simulink model "xhand_sphere_tube_r50_v3"  (R2022b)
settings: Solver=VariableStepAuto  StartTime=0.0  StopTime=5  RelTol=1e-3
InitFcn:
  | clc;
  | clear;
  | addpath('H:\研究生\新建文件夹\xhand\meshes');
  | radium=0.055
  | global flag_gravity;
  | flag_gravity=0;
undefined symbols (not defined in the file): X, Y, Z
libraries: sm_lib x125, nesl_utility x27, Contact_Forces_Lib x26
(part 4 of 5)

== system xhand_sphere_tube_r50_v3/Subsystem/t5 ==
  Inertia : sm_lib/Body Elements/Inertia  InertiaType=Custom  Mass=0.00236998990932685  MassUnits=kg  CenterOfMass=[0, 0, 0]  CenterOfMassUnits=m  MomentsOfInertia=[1.05976671520843e-07, 4.46871056730638e-08, 1.03242419674807e-07]  MomentsOfInertiaUnits=kg*m^2  ProductsOfInertia=[1.03418479605301e-08, -7.1242901669066e-14, 2.53163731637035e-13]  ProductsOfInertiaUnits=kg*m^2  GraphicType=None  MarkerShape=Inertia  MarkerSize=20  GraphicVisPropType=SimpleVisualProperties  GraphicDiffuseColor=[0.5 0.5 0.5]  GraphicSpecularColor=[0.5 0.5 0.5 1.0]  GraphicAmbientColor=[0.15 0.15 0.15 1.0]  GraphicEmissiveColor=[0.0 0.0 0.0 1.0]  GraphicShininess=75  GraphicOpacity=1.0
  InertiaOriginTransform : sm_lib/Frames and Transforms/Rigid Transform  TranslationMethod=Cartesian  TranslationStandardOffset=0  TranslationLengthUnit=m  TranslationStandardAxis=+Z  TranslationCartesianOffset=[-0.00194844009875494, 0.015770875203899, -0.00157561387804256]  TranslationROffset=0  TranslationROffsetUnits=m  TranslationZOffset=0  TranslationZOffsetUnits=m  TranslationThetaOffset=0  TranslationThetaOffsetUnits=deg  RotationMethod=RotationSequence  RotationAngleUnits=deg  RotationStandardAxis=+Z  RotationAngle=0.0  RotationArbitraryAxis=[0 0 1]  FollAlignAxisA=+X  BaseAlignAxisA=+Y  FollAlignAxisB=+Y  BaseAlignAxisB=+Z  RotationSequenceAxes=BaseAxes  RotationSequence=XYZ  RotationSequenceAngles=[0, 0, 0]  RotationSequenceAnglesUnits=rad  RotationMatrix=[1 0 0; 0 1 0; 0 0 1]  Quaternion=[1 0 0 0]
  ReferenceFrame : sm_lib/Frames and Transforms/Reference Frame
  Visual : sm_lib/Body Elements/File Solid  ExtGeomFileName=xhand/meshes/t2.STL  UnitType=Custom  ExtGeomFileUnits=m  StepReaderType=HEX  ExportConvexHullGeometry=off  InertiaType=Custom  Mass=0  MassUnits=kg  CenterOfMass=[0, 0, 0]  CenterOfMassUnits=m  MomentsOfInertia=[0, 0, 0]  MomentsOfInertiaUnits=kg*m^2  ProductsOfInertia=[0, 0, 0]  ProductsOfInertiaUnits=kg*m^2  BasedOnType=DensityFromFile  Density=1000  DensityUnits=kg/m^3  DoExposeReferenceFrame=on  SerializedFrames=<Frames/>  GraphicType=FromGeometry  MarkerShape=Sphere  MarkerSize=10  GraphicVisPropType=SimpleVisualProperties  GraphicDiffuseColor=[1, 1, 1]  GraphicSpecularColor=[0.5 0.5 0.5 1.0]  GraphicAmbientColor=[0.15 0.15 0.15 1.0]  GraphicEmissiveColor=[0.0 0.0 0.0 1.0]  GraphicShininess=75  GraphicOpacity=1
  VisualOriginTransform : sm_lib/Frames and Transforms/Rigid Transform  TranslationMethod=Cartesian  TranslationStandardOffset=0  TranslationLengthUnit=m  TranslationStandardAxis=+Z  TranslationCartesianOffset=[0, 0, 0]  TranslationROffset=0  TranslationROffsetUnits=m  TranslationZOffset=0  TranslationZOffsetUnits=m  TranslationThetaOffset=0  TranslationThetaOffsetUnits=deg  RotationMethod=RotationSequence  RotationAngleUnits=deg  RotationStandardAxis=+Z  RotationAngle=0.0  RotationArbitraryAxis=[0 0 1]  FollAlignAxisA=+X  BaseAlignAxisA=+Y  FollAlignAxisB=+Y  BaseAlignAxisB=+Z  RotationSequenceAxes=BaseAxes  RotationSequence=XYZ  RotationSequenceAngles=[0, 0, 0]  RotationSequenceAnglesUnits=rad  RotationMatrix=[1 0 0; 0 1 0; 0 0 1]  Quaternion=[1 0 0 0]
  t2_AxisInvTransform : sm_lib/Frames and Transforms/Rigid Transform  TranslationMethod=Cartesian  TranslationStandardOffset=0  TranslationLengthUnit=m  TranslationStandardAxis=+Z  TranslationCartesianOffset=[0, 0, 0]  TranslationROffset=0  TranslationROffsetUnits=m  TranslationZOffset=0  TranslationZOffsetUnits=m  TranslationThetaOffset=0  TranslationThetaOffsetUnits=deg  RotationMethod=ArbitraryAxis  RotationAngleUnits=rad  RotationStandardAxis=+Z  RotationAngle=1.570796326794897  RotationArbitraryAxis=[-0, -1, 0]  FollAlignAxisA=+X  BaseAlignAxisA=+Y  FollAlignAxisB=+Y  BaseAlignAxisB=+Z  RotationSequenceAxes=FollowerAxes  RotationSequence=XYX  RotationSequenceAngles=[0 0 0]  RotationSequenceAnglesUnits=deg  RotationMatrix=[1 0 0; 0 1 0; 0 0 1]  Quaternion=[1 0 0 0]
  F : PMIOPort  Side=Left
  t2 : PMIOPort  Port=2  Side=Left
  connections:
  Inertia/RConn1 -- InertiaOriginTransform/RConn1
  ReferenceFrame/RConn1 -- InertiaOriginTransform/LConn1 -- VisualOriginTransform/LConn1 -- t2_AxisInvTransform/LConn1
  Visual/RConn1 -- t2/RConn1 -- VisualOriginTransform/RConn1
  t2_AxisInvTransform/RConn1 -- F/RConn1

== system xhand_sphere_tube_r50_v3/Subsystem14/Subsystem10 ==
  Bus Selector10 : BusSelector  OutputSignals=Normal Force
  Bus Selector26 : BusSelector  OutputSignals=Frame Sep.x,Frame Sep.y,Frame Sep.z
  Rigid Transform10 : sm_lib/Frames and Transforms/Rigid Transform  TranslationMethod=Cartesian  TranslationStandardOffset=0  TranslationLengthUnit=m  TranslationStandardAxis=+Z  TranslationCartesianOffset=[0.0020 0.044/2 -0.000]  TranslationROffset=0  TranslationROffsetUnits=m  TranslationZOffset=0  TranslationZOffsetUnits=m  TranslationThetaOffset=0  TranslationThetaOffsetUnits=deg  RotationMethod=StandardAxis  RotationAngleUnits=deg  RotationStandardAxis=+X  RotationAngle=90.0  RotationArbitraryAxis=[0 0 1]  FollAlignAxisA=+X  BaseAlignAxisA=+Y  FollAlignAxisB=+Y  BaseAlignAxisB=+Z  RotationSequenceAxes=FollowerAxes  RotationSequence=XYX  RotationSequenceAngles=[0 0 0]  RotationSequenceAnglesUnits=deg  RotationMatrix=[1 0 0; 0 1 0; 0 0 1]  Quaternion=[1 0 0 0]
  Sphere to Plane Force7 : Contact_Forces_Lib/3D/Sphere to Plane Force  sphere_rad=0.00000000001  plane_lenx=0.00000000001  plane_leny=0.00000000001  plane_depth=0.00000000001  force_law=Nonlinear  k_contact=10e1  b_contact=10^0.5  pen_full_damp_F=1e-4  pen_exponent=1  custom_param_1=1  custom_param_2=1  friction_law=Stick-Slip Continuous  mu_kinetic=0.3  mu_static=0.5  v_thr=0.02  vis_on=on  vis_opc_en=0  vis_len_plaBz=0.0001  vis_clr=[0.9 0.2 0.2]  vis_opc=0.7
  Sphere to Tube Force8 : Contact_Forces_Lib/3D/Sphere to Tube Force  radius_sphere=radium  radius_tube=0.013/4  d_tube=0.0135/2  l_tube=0.042  active_angle=[-180 180]  force_law=Nonlinear  k_contact=1e3  b_contact=1e1  pen_full_damp_F=1e-4  pen_exponent=1  custom_param_1=1  custom_param_2=1  friction_law=Stick-Slip Continuous  mu_kinetic=0.5  mu_static=0.7  v_thr=0.001  vis_on=off  vis_opc_en=0  vis_len_tubBx=0.225*0.02  vis_clr=[0.9 0.2 0.2]  vis_opc=0.7
      settings: SourceProductName=Simscape Multibody Contact Forces Library
  mmcp : PMIOPort  Side=Right
  SphF : PMIOPort  Port=2  Side=Left
  <Normal Force> : Outport
  <x> : Outport  Port=2
  <y> : Outport  Port=3
  <z> : Outport  Port=4
  wires:
  Bus Selector26/1 -> <x>/1  "<x>"
  Bus Selector10/1 -> <Normal Force>/1  "<Normal Force>"
  Sphere to Tube Force8/1 -> Bus Selector10/1
  Sphere to Plane Force7/1 -> Bus Selector26/1
  Bus Selector26/2 -> <y>/1  "<y>"
  Bus Selector26/3 -> <z>/1  "<z>"
  connections:
  Rigid Transform10/LConn1 -- mmcp/RConn1 -- Sphere to Plane Force7/RConn1
  Sphere to Tube Force8/RConn1 -- Rigid Transform10/RConn1
  Sphere to Tube Force8/LConn1 -- Sphere to Plane Force7/LConn1 -- SphF/RConn1

== system xhand_sphere_tube_r50_v3/Subsystem14/Subsystem11 ==
  Bus Selector11 : BusSelector  OutputSignals=Normal Force
  Bus Selector39 : BusSelector  OutputSignals=Frame Sep.x,Frame Sep.y,Frame Sep.z
  Rigid Transform11 : sm_lib/Frames and Transforms/Rigid Transform  TranslationMethod=Cartesian  TranslationStandardOffset=0  TranslationLengthUnit=m  TranslationStandardAxis=+Z  TranslationCartesianOffset=[0.002 0.038/2 -0.000]  TranslationROffset=0  TranslationROffsetUnits=m  TranslationZOffset=0  TranslationZOffsetUnits=m  TranslationThetaOffset=0  TranslationThetaOffsetUnits=deg  RotationMethod=StandardAxis  RotationAngleUnits=deg  RotationStandardAxis=+X  RotationAngle=90.0  RotationArbitraryAxis=[0 0 1]  FollAlignAxisA=+X  BaseAlignAxisA=+Y  FollAlignAxisB=+Y  BaseAlignAxisB=+Z  RotationSequenceAxes=FollowerAxes  RotationSequence=XYX  RotationSequenceAngles=[0 0 0]  RotationSequenceAnglesUnits=deg  RotationMatrix=[1 0 0; 0 1 0; 0 0 1]  Quaternion=[1 0 0 0]
  Sphere to Plane Force6 : Contact_Forces_Lib/3D/Sphere to Plane Force  sphere_rad=radium+0.001  plane_lenx=0.006*2  plane_leny=0.031*2  plane_depth=0.0124/2*0.4  force_law=Nonlinear  k_contact=10e1  b_contact=10^0.5  pen_full_damp_F=1e-4  pen_exponent=1  custom_param_1=1  custom_param_2=1  friction_law=Stick-Slip Continuous  mu_kinetic=0.5  mu_static=0.7  v_thr=0.05  vis_on=off  vis_opc_en=0  vis_len_plaBz=0.0001  vis_clr=[0.9 0.2 0.2]  vis_opc=0.7
  Sphere to Tube Force9 : Contact_Forces_Lib/3D/Sphere to Tube Force  radius_sphere=radium  radius_tube=0.0135/4  d_tube=0.0135/2  l_tube=0.038  active_angle=[-180 180]  force_law=Nonlinear  k_contact=1e3  b_contact=1e1  pen_full_damp_F=1e-4  pen_exponent=1  custom_param_1=1  custom_param_2=1  friction_law=Stick-Slip Continuous  mu_kinetic=0.5  mu_static=0.7  v_thr=0.001  vis_on=off  vis_opc_en=0  vis_len_tubBx=0.225*0.02  vis_clr=[0.9 0.2 0.2]  vis_opc=0.7
      settings: SourceProductName=Simscape Multibody Contact Forces Library
  imcp : PMIOPort  Side=Right
  SphF : PMIOPort  Port=2  Side=Left
  <Normal Force> : Outport
  <x> : Outport  Port=2
  <y> : Outport  Port=3
  <z> : Outport  Port=4
  wires:
  Sphere to Tube Force9/1 -> Bus Selector11/1
  Bus Selector39/1 -> <x>/1  "<x>"
  Sphere to Plane Force6/1 -> Bus Selector39/1
  Bus Selector11/1 -> <Normal Force>/1  "<Normal Force>"
  Bus Selector39/2 -> <y>/1  "<y>"
  Bus Selector39/3 -> <z>/1  "<z>"
  connections:
  Sphere to Tube Force9/LConn1 -- Sphere to Plane Force6/LConn1 -- SphF/RConn1
  Sphere to Tube Force9/RConn1 -- Rigid Transform11/RConn1
  Rigid Transform11/LConn1 -- imcp/RConn1 -- Sphere to Plane Force6/RConn1

== system xhand_sphere_tube_r50_v3/Subsystem14/Subsystem12 ==
  Bus Selector18 : BusSelector  OutputSignals=Normal Force
  Bus Selector38 : BusSelector  OutputSignals=Frame Sep.x,Frame Sep.y,Frame Sep.z
  Rigid Transform3 : sm_lib/Frames and Transforms/Rigid Transform  TranslationMethod=Cartesian  TranslationStandardOffset=0  TranslationLengthUnit=m  TranslationStandardAxis=+Z  TranslationCartesianOffset=[0.002 0.04/2 0.0005]  TranslationROffset=0  TranslationROffsetUnits=m  TranslationZOffset=0  TranslationZOffsetUnits=m  TranslationThetaOffset=0  TranslationThetaOffsetUnits=deg  RotationMethod=StandardAxis  RotationAngleUnits=deg  RotationStandardAxis=+X  RotationAngle=90.0  RotationArbitraryAxis=[0 0 1]  FollAlignAxisA=+X  BaseAlignAxisA=+Y  FollAlignAxisB=+Y  BaseAlignAxisB=+Z  RotationSequenceAxes=FollowerAxes  RotationSequence=XYX  RotationSequenceAngles=[0 0 0]  RotationSequenceAnglesUnits=deg  RotationMatrix=[1 0 0; 0 1 0; 0 0 1]  Quaternion=[1 0 0 0]
  Sphere to Plane Force10 : Contact_Forces_Lib/3D/Sphere to Plane Force  sphere_rad=0.0000000000001  plane_lenx=0.0000000000001  plane_leny=0.0000000000001  plane_depth=0.0000000000001  force_law=Nonlinear  k_contact=10^3  b_contact=10^1  pen_full_damp_F=1e-4  pen_exponent=1  custom_param_1=1  custom_param_2=1  friction_law=Stick-Slip Continuous  mu_kinetic=0.5  mu_static=0.7  v_thr=0.05  vis_on=on  vis_opc_en=0  vis_len_plaBz=0.0001  vis_clr=[0.9 0.2 0.2]  vis_opc=0.7
  Sphere to Tube Force : Contact_Forces_Lib/3D/Sphere to Tube Force  radius_sphere=radium+0.001  radius_tube=0.0126/4  d_tube=0.0126/2  l_tube=0.033  active_angle=[-180 180]  force_law=Nonlinear  k_contact=1e3  b_contact=1e1  pen_full_damp_F=1e-4  pen_exponent=1  custom_param_1=1  custom_param_2=1  friction_law=Stick-Slip Continuous  mu_kinetic=0.5  mu_static=0.7  v_thr=0.001  vis_on=off  vis_opc_en=0  vis_len_tubBx=0.225*0.02  vis_clr=[0.9 0.2 0.2]  vis_opc=0.7
      settings: SourceProductName=Simscape Multibody Contact Forces Library
  tmcp : PMIOPort  Side=Right
  SphF : PMIOPort  Port=2  Side=Left
  <Normal Force> : Outport
  <x> : Outport  Port=2
  <y> : Outport  Port=3
  <z> : Outport  Port=4
  wires:
  Sphere to Plane Force10/1 -> Bus Selector38/1
  Sphere to Tube Force/1 -> Bus Selector18/1
  Bus Selector18/1 -> <Normal Force>/1  "<Normal Force>"
  Bus Selector38/3 -> <z>/1  "<z>"
  Bus Selector38/2 -> <y>/1  "<y>"
  Bus Selector38/1 -> <x>/1  "<x>"
  connections:
  Sphere to Tube Force/RConn1 -- Rigid Transform3/RConn1
  Rigid Transform3/LConn1 -- tmcp/RConn1 -- Sphere to Plane Force10/RConn1
  Sphere to Tube Force/LConn1 -- Sphere to Plane Force10/LConn1 -- SphF/RConn1

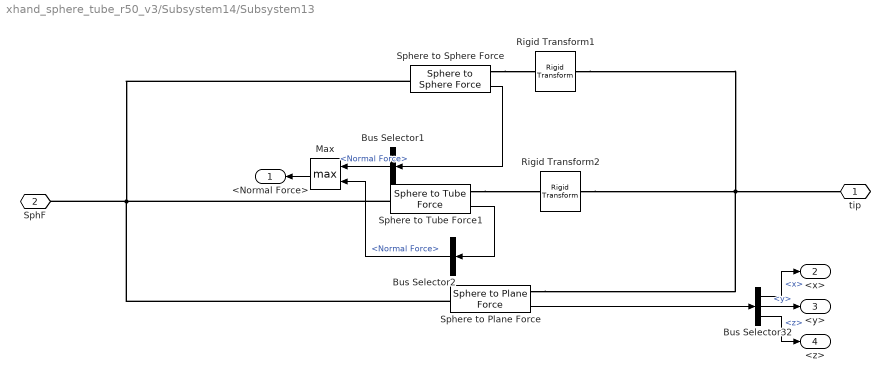
== system xhand_sphere_tube_r50_v3/Subsystem14/Subsystem13 ==
  Bus Selector1 : BusSelector  OutputSignals=Normal Force
  Bus Selector2 : BusSelector  OutputSignals=Normal Force
  Bus Selector32 : BusSelector  OutputSignals=Frame Sep.x,Frame Sep.y,Frame Sep.z
  Max : MinMax  Function=max  Inputs=2
  Rigid Transform1 : sm_lib/Frames and Transforms/Rigid Transform  TranslationMethod=Cartesian  TranslationStandardOffset=0  TranslationLengthUnit=m  TranslationStandardAxis=+Z  TranslationCartesianOffset=[-0.0019 0.053/2 -0.0022]  TranslationROffset=0  TranslationROffsetUnits=m  TranslationZOffset=0  TranslationZOffsetUnits=m  TranslationThetaOffset=0  TranslationThetaOffsetUnits=deg  RotationMethod=StandardAxis  RotationAngleUnits=deg  RotationStandardAxis=+X  RotationAngle=90.0  RotationArbitraryAxis=[0 0 1]  FollAlignAxisA=+X  BaseAlignAxisA=+Y  FollAlignAxisB=+Y  BaseAlignAxisB=+Z  RotationSequenceAxes=FollowerAxes  RotationSequence=XYX  RotationSequenceAngles=[0 0 0]  RotationSequenceAnglesUnits=deg  RotationMatrix=[1 0 0; 0 1 0; 0 0 1]  Quaternion=[1 0 0 0]
  Rigid Transform2 : sm_lib/Frames and Transforms/Rigid Transform  TranslationMethod=Cartesian  TranslationStandardOffset=0  TranslationLengthUnit=m  TranslationStandardAxis=+Z  TranslationCartesianOffset=[-0.0019 0.03/2 -0.003]  TranslationROffset=0  TranslationROffsetUnits=m  TranslationZOffset=0  TranslationZOffsetUnits=m  TranslationThetaOffset=0  TranslationThetaOffsetUnits=deg  RotationMethod=StandardAxis  RotationAngleUnits=deg  RotationStandardAxis=+X  RotationAngle=90.0  RotationArbitraryAxis=[0 0 1]  FollAlignAxisA=+X  BaseAlignAxisA=+Y  FollAlignAxisB=+Y  BaseAlignAxisB=+Z  RotationSequenceAxes=FollowerAxes  RotationSequence=XYX  RotationSequenceAngles=[0 0 0]  RotationSequenceAnglesUnits=deg  RotationMatrix=[1 0 0; 0 1 0; 0 0 1]  Quaternion=[1 0 0 0]
  Sphere to Plane Force : Contact_Forces_Lib/3D/Sphere to Plane Force  sphere_rad=0.0000000000001  plane_lenx=0.0000000000001  plane_leny=0.0000000000001  plane_depth=0.0000000000001  force_law=Nonlinear  k_contact=10^3  b_contact=10^1  pen_full_damp_F=1e-4  pen_exponent=1  custom_param_1=1  custom_param_2=1  friction_law=Stick-Slip Continuous  mu_kinetic=0.5  mu_static=0.7  v_thr=0.05  vis_on=off  vis_opc_en=0  vis_len_plaBz=0.0001  vis_clr=[0.9 0.2 0.2]  vis_opc=0.7
  Sphere to Sphere Force : Contact_Forces_Lib/3D/Sphere to Sphere Force  sphB_rad=0.0058  sphF_rad=radium  force_law=Nonlinear  k_contact=1e4  b_contact=1e2  pen_full_damp_F=1e-4  pen_exponent=1  custom_param_1=1  custom_param_2=1  friction_law=Stick-Slip Continuous  mu_kinetic=0.6  mu_static=0.7  v_thr=0.001  vis_on=off  vis_opc_en=0  vis_clr=[0.9 0.2 0.2]  vis_opc=0.7
      settings: SourceProductName=Simscape Multibody Contact Forces Library
  Sphere to Tube Force1 : Contact_Forces_Lib/3D/Sphere to Tube Force  radius_sphere=radium+0.00  radius_tube=0.012/4  d_tube=0.012/2  l_tube=0.03  active_angle=[-180 180]  force_law=Nonlinear  k_contact=1e4  b_contact=1e2  pen_full_damp_F=1e-4  pen_exponent=1  custom_param_1=1  custom_param_2=1  friction_law=Stick-Slip Continuous  mu_kinetic=0.6  mu_static=0.7  v_thr=0.001  vis_on=off  vis_opc_en=0  vis_len_tubBx=0.225*0.02  vis_clr=[0.9 0.2 0.2]  vis_opc=0.7
      settings: SourceProductName=Simscape Multibody Contact Forces Library
  tip : PMIOPort  Side=Right
  SphF : PMIOPort  Port=2  Side=Left
  <Normal Force> : Outport
  <x> : Outport  Port=2
  <y> : Outport  Port=3
  <z> : Outport  Port=4
  wires:
  Bus Selector32/1 -> <x>/1  "<x>"
  Bus Selector32/2 -> <y>/1  "<y>"
  Sphere to Plane Force/1 -> Bus Selector32/1
  Sphere to Tube Force1/1 -> Bus Selector2/1
  Bus Selector32/3 -> <z>/1  "<z>"
  Bus Selector1/1 -> Max/1  "<Normal Force>"
  Max/1 -> <Normal Force>/1
  Bus Selector2/1 -> Max/2  "<Normal Force>"
  Sphere to Sphere Force/1 -> Bus Selector1/1
  connections:
  Sphere to Tube Force1/RConn1 -- Rigid Transform2/RConn1
  Rigid Transform2/LConn1 -- Rigid Transform1/LConn1 -- tip/RConn1 -- Sphere to Plane Force/RConn1
  Sphere to Tube Force1/LConn1 -- Sphere to Sphere Force/LConn1 -- Sphere to Plane Force/LConn1 -- SphF/RConn1
  Sphere to Sphere Force/RConn1 -- Rigid Transform1/RConn1

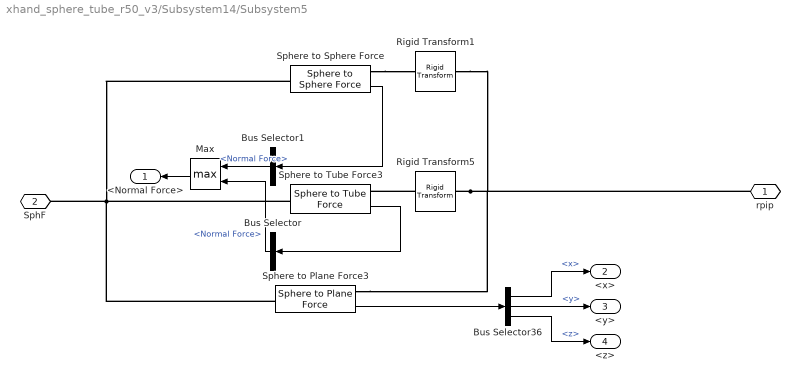
== system xhand_sphere_tube_r50_v3/Subsystem14/Subsystem5 ==
  Bus Selector : BusSelector  OutputSignals=Normal Force
  Bus Selector1 : BusSelector  OutputSignals=Normal Force
  Bus Selector36 : BusSelector  OutputSignals=Frame Sep.x,Frame Sep.y,Frame Sep.z
  Max : MinMax  Function=max  Inputs=2
  Rigid Transform1 : sm_lib/Frames and Transforms/Rigid Transform  TranslationMethod=Cartesian  TranslationStandardOffset=0  TranslationLengthUnit=m  TranslationStandardAxis=+Z  TranslationCartesianOffset=[-0.002 0.0525/2 -0.0018]  TranslationROffset=0  TranslationROffsetUnits=m  TranslationZOffset=0  TranslationZOffsetUnits=m  TranslationThetaOffset=0  TranslationThetaOffsetUnits=deg  RotationMethod=StandardAxis  RotationAngleUnits=deg  RotationStandardAxis=+X  RotationAngle=90.0  RotationArbitraryAxis=[0 0 1]  FollAlignAxisA=+X  BaseAlignAxisA=+Y  FollAlignAxisB=+Y  BaseAlignAxisB=+Z  RotationSequenceAxes=FollowerAxes  RotationSequence=XYX  RotationSequenceAngles=[0 0 0]  RotationSequenceAnglesUnits=deg  RotationMatrix=[1 0 0; 0 1 0; 0 0 1]  Quaternion=[1 0 0 0]
  Rigid Transform5 : sm_lib/Frames and Transforms/Rigid Transform  TranslationMethod=Cartesian  TranslationStandardOffset=0  TranslationLengthUnit=m  TranslationStandardAxis=+Z  TranslationCartesianOffset=[-0.0019 0.032/2 -0.0018]  TranslationROffset=0  TranslationROffsetUnits=m  TranslationZOffset=0  TranslationZOffsetUnits=m  TranslationThetaOffset=0  TranslationThetaOffsetUnits=deg  RotationMethod=StandardAxis  RotationAngleUnits=deg  RotationStandardAxis=+X  RotationAngle=90.0  RotationArbitraryAxis=[0 0 1]  FollAlignAxisA=+X  BaseAlignAxisA=+Y  FollAlignAxisB=+Y  BaseAlignAxisB=+Z  RotationSequenceAxes=FollowerAxes  RotationSequence=XYX  RotationSequenceAngles=[0 0 0]  RotationSequenceAnglesUnits=deg  RotationMatrix=[1 0 0; 0 1 0; 0 0 1]  Quaternion=[1 0 0 0]
  Sphere to Plane Force3 : Contact_Forces_Lib/3D/Sphere to Plane Force  sphere_rad=0.00000000001  plane_lenx=0.00000000001  plane_leny=0.00000000001  plane_depth=0.00000000001  force_law=Nonlinear  k_contact=10e1  b_contact=10^0.5  pen_full_damp_F=1e-4  pen_exponent=1  custom_param_1=1  custom_param_2=1  friction_law=Stick-Slip Continuous  mu_kinetic=0.5  mu_static=0.7  v_thr=0.05  vis_on=off  vis_opc_en=0  vis_len_plaBz=0.0001  vis_clr=[0.9 0.2 0.2]  vis_opc=0.7
  Sphere to Sphere Force : Contact_Forces_Lib/3D/Sphere to Sphere Force  sphB_rad=0.006  sphF_rad=radium  force_law=Nonlinear  k_contact=1e4  b_contact=1e2  pen_full_damp_F=1e-4  pen_exponent=1  custom_param_1=1  custom_param_2=1  friction_law=Stick-Slip Continuous  mu_kinetic=0.6  mu_static=0.7  v_thr=0.001  vis_on=off  vis_opc_en=0  vis_clr=[0.9 0.2 0.2]  vis_opc=0.7
      settings: SourceProductName=Simscape Multibody Contact Forces Library
  Sphere to Tube Force3 : Contact_Forces_Lib/3D/Sphere to Tube Force  radius_sphere=radium  radius_tube=0.011/4  d_tube=0.012/2  l_tube=0.032  active_angle=[-180 180]  force_law=Nonlinear  k_contact=1e4  b_contact=1e2  pen_full_damp_F=1e-4  pen_exponent=1  custom_param_1=1  custom_param_2=1  friction_law=Stick-Slip Continuous  mu_kinetic=0.6  mu_static=0.7  v_thr=0.001  vis_on=off  vis_opc_en=0  vis_len_tubBx=0.225*0.02  vis_clr=[0.9 0.2 0.2]  vis_opc=0.7
      settings: SourceProductName=Simscape Multibody Contact Forces Library
  rpip : PMIOPort  Side=Right
  SphF : PMIOPort  Port=2  Side=Left
  <Normal Force> : Outport
  <x> : Outport  Port=2
  <y> : Outport  Port=3
  <z> : Outport  Port=4
  wires:
  Sphere to Tube Force3/1 -> Bus Selector/1
  Sphere to Plane Force3/1 -> Bus Selector36/1
  Bus Selector36/2 -> <y>/1  "<y>"
  Bus Selector36/3 -> <z>/1  "<z>"
  Bus Selector36/1 -> <x>/1  "<x>"
  Sphere to Sphere Force/1 -> Bus Selector1/1
  Max/1 -> <Normal Force>/1
  Bus Selector/1 -> Max/2  "<Normal Force>"
  Bus Selector1/1 -> Max/1  "<Normal Force>"
  connections:
  Rigid Transform5/LConn1 -- Rigid Transform1/LConn1 -- rpip/RConn1 -- Sphere to Plane Force3/RConn1
  Rigid Transform5/RConn1 -- Sphere to Tube Force3/RConn1
  Sphere to Tube Force3/LConn1 -- Sphere to Sphere Force/LConn1 -- Sphere to Plane Force3/LConn1 -- SphF/RConn1
  Sphere to Sphere Force/RConn1 -- Rigid Transform1/RConn1

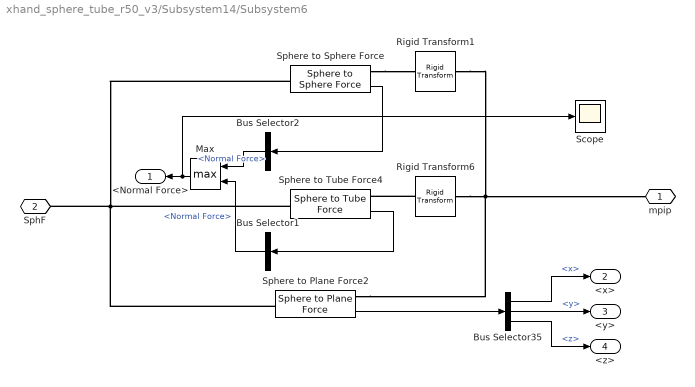
== system xhand_sphere_tube_r50_v3/Subsystem14/Subsystem6 ==
  Bus Selector1 : BusSelector  OutputSignals=Normal Force
  Bus Selector2 : BusSelector  OutputSignals=Normal Force
  Bus Selector35 : BusSelector  OutputSignals=Frame Sep.x,Frame Sep.y,Frame Sep.z
  Max : MinMax  Function=max  Inputs=2
  Rigid Transform1 : sm_lib/Frames and Transforms/Rigid Transform  TranslationMethod=Cartesian  TranslationStandardOffset=0  TranslationLengthUnit=m  TranslationStandardAxis=+Z  TranslationCartesianOffset=[-0.0019 0.0705/2 -0.0019]  TranslationROffset=0  TranslationROffsetUnits=m  TranslationZOffset=0  TranslationZOffsetUnits=m  TranslationThetaOffset=0  TranslationThetaOffsetUnits=deg  RotationMethod=StandardAxis  RotationAngleUnits=deg  RotationStandardAxis=+X  RotationAngle=90.0  RotationArbitraryAxis=[0 0 1]  FollAlignAxisA=+X  BaseAlignAxisA=+Y  FollAlignAxisB=+Y  BaseAlignAxisB=+Z  RotationSequenceAxes=FollowerAxes  RotationSequence=XYX  RotationSequenceAngles=[0 0 0]  RotationSequenceAnglesUnits=deg  RotationMatrix=[1 0 0; 0 1 0; 0 0 1]  Quaternion=[1 0 0 0]
  Rigid Transform6 : sm_lib/Frames and Transforms/Rigid Transform  TranslationMethod=Cartesian  TranslationStandardOffset=0  TranslationLengthUnit=m  TranslationStandardAxis=+Z  TranslationCartesianOffset=[-0.0019 0.038/2 -0.0018]  TranslationROffset=0  TranslationROffsetUnits=m  TranslationZOffset=0  TranslationZOffsetUnits=m  TranslationThetaOffset=0  TranslationThetaOffsetUnits=deg  RotationMethod=StandardAxis  RotationAngleUnits=deg  RotationStandardAxis=+X  RotationAngle=90.0  RotationArbitraryAxis=[0 0 1]  FollAlignAxisA=+X  BaseAlignAxisA=+Y  FollAlignAxisB=+Y  BaseAlignAxisB=+Z  RotationSequenceAxes=FollowerAxes  RotationSequence=XYX  RotationSequenceAngles=[0 0 0]  RotationSequenceAnglesUnits=deg  RotationMatrix=[1 0 0; 0 1 0; 0 0 1]  Quaternion=[1 0 0 0]
  Scope : Scope
  Sphere to Plane Force2 : Contact_Forces_Lib/3D/Sphere to Plane Force  sphere_rad=0.00000000001  plane_lenx=0.00000000001  plane_leny=0.00000000001  plane_depth=0.00000000001  force_law=Nonlinear  k_contact=10e3  b_contact=10^1  pen_full_damp_F=1e-4  pen_exponent=1  custom_param_1=1  custom_param_2=1  friction_law=Stick-Slip Continuous  mu_kinetic=0.3  mu_static=0.5  v_thr=0.02  vis_on=off  vis_opc_en=0  vis_len_plaBz=0.0001  vis_clr=[0.9 0.2 0.2]  vis_opc=0.7
  Sphere to Sphere Force : Contact_Forces_Lib/3D/Sphere to Sphere Force  sphB_rad=0.0053  sphF_rad=radium  force_law=Nonlinear  k_contact=1e4  b_contact=1e2  pen_full_damp_F=1e-4  pen_exponent=1  custom_param_1=1  custom_param_2=1  friction_law=Stick-Slip Continuous  mu_kinetic=0.6  mu_static=0.7  v_thr=0.001  vis_on=off  vis_opc_en=0  vis_clr=[0.9 0.2 0.2]  vis_opc=0.7
      settings: SourceProductName=Simscape Multibody Contact Forces Library
  Sphere to Tube Force4 : Contact_Forces_Lib/3D/Sphere to Tube Force  radius_sphere=radium+0.00  radius_tube=0.0118/4  d_tube=0.01/2  l_tube=0.04  active_angle=[-180 180]  force_law=Nonlinear  k_contact=1e4  b_contact=1e2  pen_full_damp_F=1e-4  pen_exponent=1  custom_param_1=1  custom_param_2=1  friction_law=Stick-Slip Continuous  mu_kinetic=0.6  mu_static=0.7  v_thr=0.001  vis_on=off  vis_opc_en=0  vis_len_tubBx=0.225*0.02  vis_clr=[0.9 0.2 0.2]  vis_opc=0.7
      settings: SourceProductName=Simscape Multibody Contact Forces Library
  mpip : PMIOPort  Side=Right
  SphF : PMIOPort  Port=2  Side=Left
  <Normal Force> : Outport
  <x> : Outport  Port=2
  <y> : Outport  Port=3
  <z> : Outport  Port=4
  wires:
  Sphere to Plane Force2/1 -> Bus Selector35/1
  Sphere to Tube Force4/1 -> Bus Selector1/1
  Bus Selector35/2 -> <y>/1  "<y>"
  Bus Selector35/1 -> <x>/1  "<x>"
  Bus Selector35/3 -> <z>/1  "<z>"
  Sphere to Sphere Force/1 -> Bus Selector2/1
  Max/1 -> Scope/1, <Normal Force>/1
  Bus Selector1/1 -> Max/2  "<Normal Force>"
  Bus Selector2/1 -> Max/1  "<Normal Force>"
  connections:
  Sphere to Tube Force4/LConn1 -- Sphere to Plane Force2/LConn1 -- Sphere to Sphere Force/LConn1 -- SphF/RConn1
  Rigid Transform6/LConn1 -- Rigid Transform1/LConn1 -- mpip/RConn1 -- Sphere to Plane Force2/RConn1
  Rigid Transform6/RConn1 -- Sphere to Tube Force4/RConn1
  Sphere to Sphere Force/RConn1 -- Rigid Transform1/RConn1

== system xhand_sphere_tube_r50_v3/Subsystem14/Subsystem7 ==
  Bus Selector1 : BusSelector  OutputSignals=Normal Force
  Bus Selector29 : BusSelector  OutputSignals=Frame Sep.x,Frame Sep.y,Frame Sep.z
  Bus Selector3 : BusSelector  OutputSignals=Normal Force
  Max : MinMax  Function=max  Inputs=2
  Rigid Transform1 : sm_lib/Frames and Transforms/Rigid Transform  TranslationMethod=Cartesian  TranslationStandardOffset=0  TranslationLengthUnit=m  TranslationStandardAxis=+Z  TranslationCartesianOffset=[-0.0021 0.049/2 -0.0023]  TranslationROffset=0  TranslationROffsetUnits=m  TranslationZOffset=0  TranslationZOffsetUnits=m  TranslationThetaOffset=0  TranslationThetaOffsetUnits=deg  RotationMethod=StandardAxis  RotationAngleUnits=deg  RotationStandardAxis=+X  RotationAngle=90.0  RotationArbitraryAxis=[0 0 1]  FollAlignAxisA=+X  BaseAlignAxisA=+Y  FollAlignAxisB=+Y  BaseAlignAxisB=+Z  RotationSequenceAxes=FollowerAxes  RotationSequence=XYX  RotationSequenceAngles=[0 0 0]  RotationSequenceAnglesUnits=deg  RotationMatrix=[1 0 0; 0 1 0; 0 0 1]  Quaternion=[1 0 0 0]
  Rigid Transform7 : sm_lib/Frames and Transforms/Rigid Transform  TranslationMethod=Cartesian  TranslationStandardOffset=0  TranslationLengthUnit=m  TranslationStandardAxis=+Z  TranslationCartesianOffset=[-0.0021 0.030/2 -0.002]  TranslationROffset=0  TranslationROffsetUnits=m  TranslationZOffset=0  TranslationZOffsetUnits=m  TranslationThetaOffset=0  TranslationThetaOffsetUnits=deg  RotationMethod=StandardAxis  RotationAngleUnits=deg  RotationStandardAxis=+X  RotationAngle=90.0  RotationArbitraryAxis=[0 0 1]  FollAlignAxisA=+X  BaseAlignAxisA=+Y  FollAlignAxisB=+Y  BaseAlignAxisB=+Z  RotationSequenceAxes=FollowerAxes  RotationSequence=XYX  RotationSequenceAngles=[0 0 0]  RotationSequenceAnglesUnits=deg  RotationMatrix=[1 0 0; 0 1 0; 0 0 1]  Quaternion=[1 0 0 0]
  Sphere to Plane Force1 : Contact_Forces_Lib/3D/Sphere to Plane Force  sphere_rad=0.00000000001  plane_lenx=0.00000000001  plane_leny=0.00000000001  plane_depth=0.00000000001  force_law=Nonlinear  k_contact=10e1  b_contact=10^0.5  pen_full_damp_F=1e-4  pen_exponent=1  custom_param_1=1  custom_param_2=1  friction_law=Stick-Slip Continuous  mu_kinetic=0.5  mu_static=0.7  v_thr=0.05  vis_on=off  vis_opc_en=0  vis_len_plaBz=0.0001  vis_clr=[0.9 0.2 0.2]  vis_opc=0.7
  Sphere to Sphere Force : Contact_Forces_Lib/3D/Sphere to Sphere Force  sphB_rad=0.0058  sphF_rad=radium  force_law=Nonlinear  k_contact=1e4  b_contact=1e2  pen_full_damp_F=1e-4  pen_exponent=1  custom_param_1=1  custom_param_2=1  friction_law=Stick-Slip Continuous  mu_kinetic=0.6  mu_static=0.7  v_thr=0.001  vis_on=off  vis_opc_en=0  vis_clr=[0.9 0.2 0.2]  vis_opc=0.7
      settings: SourceProductName=Simscape Multibody Contact Forces Library
  Sphere to Tube Force5 : Contact_Forces_Lib/3D/Sphere to Tube Force  radius_sphere=radium  radius_tube=0.012/4  d_tube=0.012/2  l_tube=0.03  active_angle=[-180 180]  force_law=Nonlinear  k_contact=1e4  b_contact=1e2  pen_full_damp_F=1e-4  pen_exponent=1  custom_param_1=1  custom_param_2=1  friction_law=Stick-Slip Continuous  mu_kinetic=0.6  mu_static=0.7  v_thr=0.001  vis_on=off  vis_opc_en=0  vis_len_tubBx=0.225*0.02  vis_clr=[0.9 0.2 0.2]  vis_opc=0.7
      settings: SourceProductName=Simscape Multibody Contact Forces Library
  ipip : PMIOPort  Side=Right
  SphF : PMIOPort  Port=2  Side=Left
  <Normal Force> : Outport
  <x> : Outport  Port=2
  <y> : Outport  Port=3
  <z> : Outport  Port=4
  wires:
  Sphere to Tube Force5/1 -> Bus Selector3/1
  Sphere to Plane Force1/1 -> Bus Selector29/1
  Bus Selector3/1 -> Max/2  "<Normal Force>"
  Bus Selector29/3 -> <z>/1  "<z>"
  Bus Selector29/2 -> <y>/1  "<y>"
  Bus Selector29/1 -> <x>/1  "<x>"
  Sphere to Sphere Force/1 -> Bus Selector1/1
  Bus Selector1/1 -> Max/1  "<Normal Force>"
  Max/1 -> <Normal Force>/1
  connections:
  Sphere to Tube Force5/LConn1 -- Sphere to Plane Force1/LConn1 -- Sphere to Sphere Force/LConn1 -- SphF/RConn1
  Rigid Transform7/RConn1 -- Sphere to Tube Force5/RConn1
  ipip/RConn1 -- Rigid Transform1/LConn1 -- Sphere to Plane Force1/RConn1 -- Rigid Transform7/LConn1
  Sphere to Sphere Force/RConn1 -- Rigid Transform1/RConn1

== system xhand_sphere_tube_r50_v3/Subsystem14/Subsystem8 ==
  Bus Selector13 : BusSelector  OutputSignals=Normal Force
  Bus Selector28 : BusSelector  OutputSignals=Frame Sep.x,Frame Sep.y,Frame Sep.z
  Rigid Transform8 : sm_lib/Frames and Transforms/Rigid Transform  TranslationMethod=Cartesian  TranslationStandardOffset=0  TranslationLengthUnit=m  TranslationStandardAxis=+Z  TranslationCartesianOffset=[0.0020 0.030/2 -0.000]  TranslationROffset=0  TranslationROffsetUnits=m  TranslationZOffset=0  TranslationZOffsetUnits=m  TranslationThetaOffset=0  TranslationThetaOffsetUnits=deg  RotationMethod=StandardAxis  RotationAngleUnits=deg  RotationStandardAxis=+X  RotationAngle=90.0  RotationArbitraryAxis=[0 0 1]  FollAlignAxisA=+X  BaseAlignAxisA=+Y  FollAlignAxisB=+Y  BaseAlignAxisB=+Z  RotationSequenceAxes=FollowerAxes  RotationSequence=XYX  RotationSequenceAngles=[0 0 0]  RotationSequenceAnglesUnits=deg  RotationMatrix=[1 0 0; 0 1 0; 0 0 1]  Quaternion=[1 0 0 0]
  Sphere to Plane Force9 : Contact_Forces_Lib/3D/Sphere to Plane Force  sphere_rad=0.00000000001  plane_lenx=0.00000000001  plane_leny=0.00000000001  plane_depth=0.00000000001  force_law=Nonlinear  k_contact=10e1  b_contact=10^0.5  pen_full_damp_F=1e-4  pen_exponent=1  custom_param_1=1  custom_param_2=1  friction_law=Stick-Slip Continuous  mu_kinetic=0.5  mu_static=0.7  v_thr=0.05  vis_on=off  vis_opc_en=0  vis_len_plaBz=0.0001  vis_clr=[0.9 0.2 0.2]  vis_opc=0.7
  Sphere to Tube Force6 : Contact_Forces_Lib/3D/Sphere to Tube Force  radius_sphere=radium  radius_tube=0.0135/4  d_tube=0.0135/2  l_tube=0.03  active_angle=[-180 180]  force_law=Nonlinear  k_contact=1e3  b_contact=1e1  pen_full_damp_F=1e-4  pen_exponent=1  custom_param_1=1  custom_param_2=1  friction_law=Stick-Slip Continuous  mu_kinetic=0.5  mu_static=0.7  v_thr=0.001  vis_on=off  vis_opc_en=0  vis_len_tubBx=0.225*0.02  vis_clr=[0.9 0.2 0.2]  vis_opc=0.7
      settings: SourceProductName=Simscape Multibody Contact Forces Library
  lmcp : PMIOPort  Side=Right
  SphF : PMIOPort  Port=2  Side=Left
  <Normal Force> : Outport
  <x> : Outport  Port=2
  <y> : Outport  Port=3
  <z> : Outport  Port=4
  wires:
  Sphere to Tube Force6/1 -> Bus Selector13/1
  Sphere to Plane Force9/1 -> Bus Selector28/1
  Bus Selector13/1 -> <Normal Force>/1  "<Normal Force>"
  Bus Selector28/1 -> <x>/1  "<x>"
  Bus Selector28/2 -> <y>/1  "<y>"
  Bus Selector28/3 -> <z>/1  "<z>"
  connections:
  Sphere to Tube Force6/LConn1 -- Sphere to Plane Force9/LConn1 -- SphF/RConn1
  Sphere to Tube Force6/RConn1 -- Rigid Transform8/RConn1
  Rigid Transform8/LConn1 -- Sphere to Plane Force9/RConn1 -- lmcp/RConn1

== system xhand_sphere_tube_r50_v3/Subsystem14/Subsystem9 ==
  Bus Selector12 : BusSelector  OutputSignals=Normal Force
  Bus Selector27 : BusSelector  OutputSignals=Frame Sep.x,Frame Sep.y,Frame Sep.z
  Rigid Transform9 : sm_lib/Frames and Transforms/Rigid Transform  TranslationMethod=Cartesian  TranslationStandardOffset=0  TranslationLengthUnit=m  TranslationStandardAxis=+Z  TranslationCartesianOffset=[0.0020 0.042/2 -0.000]  TranslationROffset=0  TranslationROffsetUnits=m  TranslationZOffset=0  TranslationZOffsetUnits=m  TranslationThetaOffset=0  TranslationThetaOffsetUnits=deg  RotationMethod=StandardAxis  RotationAngleUnits=deg  RotationStandardAxis=+X  RotationAngle=90.0  RotationArbitraryAxis=[0 0 1]  FollAlignAxisA=+X  BaseAlignAxisA=+Y  FollAlignAxisB=+Y  BaseAlignAxisB=+Z  RotationSequenceAxes=FollowerAxes  RotationSequence=XYX  RotationSequenceAngles=[0 0 0]  RotationSequenceAnglesUnits=deg  RotationMatrix=[1 0 0; 0 1 0; 0 0 1]  Quaternion=[1 0 0 0]
  Sphere to Plane Force8 : Contact_Forces_Lib/3D/Sphere to Plane Force  sphere_rad=0.00000000001  plane_lenx=0.00000000001  plane_leny=0.00000000001  plane_depth=0.00000000001  force_law=Nonlinear  k_contact=10e1  b_contact=10^0.5  pen_full_damp_F=1e-4  pen_exponent=1  custom_param_1=1  custom_param_2=1  friction_law=Stick-Slip Continuous  mu_kinetic=0.5  mu_static=0.7  v_thr=0.05  vis_on=off  vis_opc_en=0  vis_len_plaBz=0.0001  vis_clr=[0.9 0.2 0.2]  vis_opc=0.7
  Sphere to Tube Force7 : Contact_Forces_Lib/3D/Sphere to Tube Force  radius_sphere=radium  radius_tube=0.0135/4  d_tube=0.0135/2  l_tube=0.04  active_angle=[-180 180]  force_law=Nonlinear  k_contact=1e3  b_contact=1e1  pen_full_damp_F=1e-4  pen_exponent=1  custom_param_1=1  custom_param_2=1  friction_law=Stick-Slip Continuous  mu_kinetic=0.5  mu_static=0.7  v_thr=0.001  vis_on=off  vis_opc_en=0  vis_len_tubBx=0.225*0.02  vis_clr=[0.9 0.2 0.2]  vis_opc=0.7
      settings: SourceProductName=Simscape Multibody Contact Forces Library
  rmcp : PMIOPort  Side=Right
  SphF : PMIOPort  Port=2  Side=Left
  <Normal Force> : Outport
  <x> : Outport  Port=2
  <y> : Outport  Port=3
  <z> : Outport  Port=4
  wires:
  Sphere to Plane Force8/1 -> Bus Selector27/1
  Bus Selector27/3 -> <z>/1  "<z>"
  Sphere to Tube Force7/1 -> Bus Selector12/1
  Bus Selector12/1 -> <Normal Force>/1  "<Normal Force>"
  Bus Selector27/2 -> <y>/1  "<y>"
  Bus Selector27/1 -> <x>/1  "<x>"
  connections:
  Sphere to Tube Force7/RConn1 -- Rigid Transform9/RConn1
  Sphere to Tube Force7/LConn1 -- Sphere to Plane Force8/LConn1 -- SphF/RConn1
  Rigid Transform9/LConn1 -- rmcp/RConn1 -- Sphere to Plane Force8/RConn1

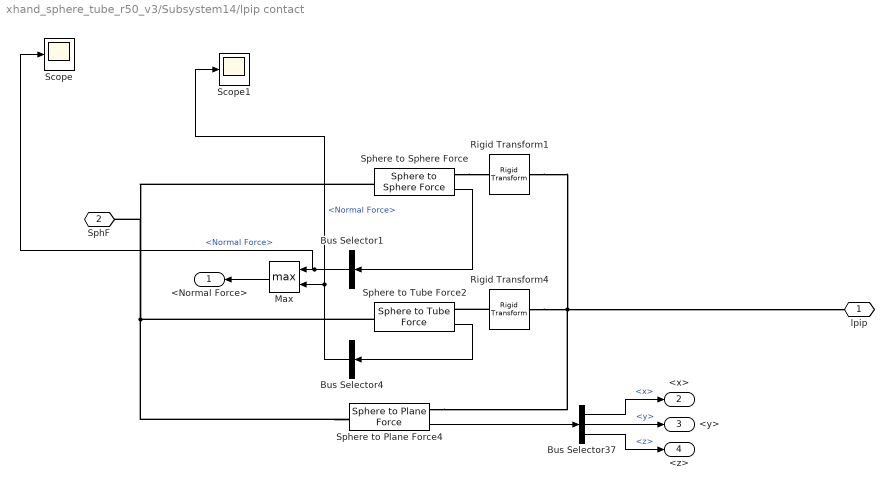
== system xhand_sphere_tube_r50_v3/Subsystem14/lpip contact ==
  Bus Selector1 : BusSelector  OutputSignals=Normal Force
  Bus Selector37 : BusSelector  OutputSignals=Frame Sep.x,Frame Sep.y,Frame Sep.z
  Bus Selector4 : BusSelector  OutputSignals=Normal Force
  Max : MinMax  Function=max  Inputs=2
  Rigid Transform1 : sm_lib/Frames and Transforms/Rigid Transform  TranslationMethod=Cartesian  TranslationStandardOffset=0  TranslationLengthUnit=m  TranslationStandardAxis=+Z  TranslationCartesianOffset=[-0.0021 0.047/2 -0.0023]  TranslationROffset=0  TranslationROffsetUnits=m  TranslationZOffset=0  TranslationZOffsetUnits=m  TranslationThetaOffset=0  TranslationThetaOffsetUnits=deg  RotationMethod=StandardAxis  RotationAngleUnits=deg  RotationStandardAxis=+X  RotationAngle=90.0  RotationArbitraryAxis=[0 0 1]  FollAlignAxisA=+X  BaseAlignAxisA=+Y  FollAlignAxisB=+Y  BaseAlignAxisB=+Z  RotationSequenceAxes=FollowerAxes  RotationSequence=XYX  RotationSequenceAngles=[0 0 0]  RotationSequenceAnglesUnits=deg  RotationMatrix=[1 0 0; 0 1 0; 0 0 1]  Quaternion=[1 0 0 0]
  Rigid Transform4 : sm_lib/Frames and Transforms/Rigid Transform  TranslationMethod=Cartesian  TranslationStandardOffset=0  TranslationLengthUnit=m  TranslationStandardAxis=+Z  TranslationCartesianOffset=[-0.0019 0.03/2 -0.002]  TranslationROffset=0  TranslationROffsetUnits=m  TranslationZOffset=0  TranslationZOffsetUnits=m  TranslationThetaOffset=0  TranslationThetaOffsetUnits=deg  RotationMethod=StandardAxis  RotationAngleUnits=deg  RotationStandardAxis=+X  RotationAngle=90.0  RotationArbitraryAxis=[0 0 1]  FollAlignAxisA=+X  BaseAlignAxisA=+Y  FollAlignAxisB=+Y  BaseAlignAxisB=+Z  RotationSequenceAxes=FollowerAxes  RotationSequence=XYX  RotationSequenceAngles=[0 0 0]  RotationSequenceAnglesUnits=deg  RotationMatrix=[1 0 0; 0 1 0; 0 0 1]  Quaternion=[1 0 0 0]
  Scope : Scope
  Scope1 : Scope
  Sphere to Plane Force4 : Contact_Forces_Lib/3D/Sphere to Plane Force  sphere_rad=0.00000000001  plane_lenx=0.00000000001  plane_leny=0.00000000001  plane_depth=0.00000000001  force_law=Nonlinear  k_contact=10e1  b_contact=10^0.5  pen_full_damp_F=1e-4  pen_exponent=1  custom_param_1=1  custom_param_2=1  friction_law=Stick-Slip Continuous  mu_kinetic=0.5  mu_static=0.7  v_thr=0.05  vis_on=on  vis_opc_en=0  vis_len_plaBz=0.0001  vis_clr=[0.9 0.2 0.2]  vis_opc=0.7
  Sphere to Sphere Force : Contact_Forces_Lib/3D/Sphere to Sphere Force  sphB_rad=0.0057  sphF_rad=radium  force_law=Nonlinear  k_contact=1e4  b_contact=1e2  pen_full_damp_F=1e-4  pen_exponent=1  custom_param_1=1  custom_param_2=1  friction_law=Stick-Slip Continuous  mu_kinetic=0.6  mu_static=0.7  v_thr=0.001  vis_on=off  vis_opc_en=0  vis_clr=[0.9 0.2 0.2]  vis_opc=0.7
      settings: SourceProductName=Simscape Multibody Contact Forces Library
  Sphere to Tube Force2 : Contact_Forces_Lib/3D/Sphere to Tube Force  radius_sphere=radium  radius_tube=0.0105/4  d_tube=0.011/2  l_tube=0.028  active_angle=[-180 180]  force_law=Nonlinear  k_contact=1e4  b_contact=1e2  pen_full_damp_F=1e-4  pen_exponent=1  custom_param_1=1  custom_param_2=1  friction_law=Stick-Slip Continuous  mu_kinetic=0.6  mu_static=0.7  v_thr=0.001  vis_on=off  vis_opc_en=0  vis_len_tubBx=0.225*0.02  vis_clr=[0.9 0.2 0.2]  vis_opc=0.7
      settings: SourceProductName=Simscape Multibody Contact Forces Library
  lpip : PMIOPort  Side=Right
  SphF : PMIOPort  Port=2  Side=Left
  <Normal Force> : Outport
  <x> : Outport  Port=2
  <y> : Outport  Port=3
  <z> : Outport  Port=4
  wires:
  Sphere to Plane Force4/1 -> Bus Selector37/1
  Bus Selector37/1 -> <x>/1  "<x>"
  Sphere to Tube Force2/1 -> Bus Selector4/1
  Bus Selector37/2 -> <y>/1  "<y>"
  Bus Selector37/3 -> <z>/1  "<z>"
  Sphere to Sphere Force/1 -> Bus Selector1/1
  Bus Selector1/1 -> Scope/1, Max/1  "<Normal Force>"
  Max/1 -> <Normal Force>/1
  Bus Selector4/1 -> Scope1/1, Max/2  "<Normal Force>"
  connections:
  Sphere to Plane Force4/LConn1 -- Sphere to Sphere Force/LConn1 -- SphF/RConn1 -- Sphere to Tube Force2/LConn1
  Sphere to Plane Force4/RConn1 -- Rigid Transform1/LConn1 -- lpip/RConn1 -- Rigid Transform4/LConn1
  Rigid Transform4/RConn1 -- Sphere to Tube Force2/RConn1
  Sphere to Sphere Force/RConn1 -- Rigid Transform1/RConn1

== matlab function xhand_sphere_tube_r50_v3/contact position rpip ==
  data: x input; xx output; y input; z input; q1 input; q2 input; yy output; zz output; l output
function [xx,yy,zz,l] = fcn(x,y,z,q1,q2)

%在食指坐标系下的坐标值
xx1=0+x;
yy1=37.77*cos(q1)+y*cos(q1+q2);
zz=37.77*sin(q1)+y*cos(q1+q2);

%在与中指坐标系的平行系下的坐标值
alpha=atan(yy1/xx1);
l=norm([xx1,yy1]);
xx2=l*cos(alpha+3.5*pi/180);
yy2=l*sin(alpha+3.5*pi/180);

%在种植坐标系下的坐标值
xx=xx2-15.9255*cos(3.5*pi/180)-1.2;
yy=yy2-15.9255*sin(3.5*pi/180)+7.5;
zz=zz+8.5;

l=z;

== matlab function xhand_sphere_tube_r50_v3/contact position lpip ==
  data: x input; xx output; y input; z input; q1 input; q2 input; yy output; zz output; l output
function [xx,yy,zz,l] = fcn(x,y,z,q1,q2)

%在食指坐标系下的坐标值
xx1=0+x;
yy1=27.77*cos(q1)+y*cos(q1+q2);
zz=27.77*sin(q1)+y*cos(q1+q2);

%在与中指坐标系的平行系下的坐标值
alpha=atan(yy1/xx1);
l=norm([xx1,yy1]);
xx2=l*cos(alpha+7*pi/180);
yy2=l*sin(alpha+7*pi/180);

%在种植坐标系下的坐标值
xx=xx2-38.4871*cos(7*pi/180)-1.2;
yy=yy2-38.4871*sin(7*pi/180)+7.5;
zz=zz+8.5;

l=z;

== matlab function xhand_sphere_tube_r50_v3/MATLAB Function6 ==
  data: f1 input; y output; f2 input; v1 input; v2 input; j input size=[6,4]
function y = fcn(f1,f2,v1,v2,j)
t=[f1*v1/norm(v1) f2*v2/norm(v2)]*j;
y=abs(t(1))+abs(t(2));

== matlab function xhand_sphere_tube_r50_v3/MATLAB Function4 ==
  data: x0 input; v1 output; y0 input; z0 input; x1 input; y1 input; z1 input; x2 input; y2 input; z2 input; v2 output
function [v1,v2] = fcn(x0,y0,z0,x1,y1,z1,x2,y2,z2)
v1=[x1-x0,y1-y0,z1-z0];
v2=[x2-x0,y2-y0,z2-z0];

== matlab function xhand_sphere_tube_r50_v3/contact position tmcp  ==
  data: x input; xx output; y input; q1 input; q2 input; yy output; zz output; q3 input
function [xx,yy,zz] = fcn(x,y,q1,q2,q3)
l01=36.17; l02=18.0;
theta01=45*3.14/180;    %初始位置和xz平面夹角
theta02=15*3.14/180;    %初始位置和xy平面夹角
trans0=[l01*cos(q2+theta01)+y*cos(q2+q3+theta01) l01*sin(q2+theta01)+y*sin(q2+q3+theta01) x 1];
p011=[19.35 -59.86 24.22 1]; p012=[15.18 -55.55 24.40 1];   %大拇指侧摆位置两点
p01=(p011+p012)/2;  p01(4)=1;
direction=[1 -1 0 1];
p021=[26.41 -44.30 24.60 1]; p022=[25.97 -44.85 27.52 1];   %大拇指近指滑轮两点
p02=(p021+p022)/2; p02(4)=1;
a1x=abs(atan(direction(2)/direction(3)));
a1y=abs(atan(direction(1)/(direction(2)^2+direction(3)^2)^0.5));
position01=p02*[[1 0 0 0]' [0 1 0 0]' [0 0 1 0]' [-p01(1) -p01(2) -p01(3) 1]']'...
    *[[1 0 0 0]' [0 cos(a1x) sin(a1x) 0]' [0 -sin(a1x) cos(a1x) 0]' [0 0 0 1]']'*[[cos(a1y) 0 -sin(a1y) 0]' [0 1 0 0]'  [sin(a1y) 0 cos(a1y) 0]' [0 0 0 1]']'...
    *[[cos(theta02) sin(theta02) 0 0]' [-sin(theta02) cos(theta02) 0 0]' [0 0 1 0]' [0 0 0 1]']'...
    *[[cos(-a1y) 0 -sin(-a1y) 0]' [0 1 0 0]'  [sin(-a1y) 0 cos(-a1y) 0]' [0 0 0 1]']'*[[1 0 0 0]' [0 cos(-a1x) sin(-a1x) 0]' [0 -sin(-a1x) cos(-a1x) 0]' [0 0 0 1]']'...
    *[[1 0 0 0]' [0 1 0 0]' [0 0 1 0]' [p01(1) p01(2) p01(3) 1]']';
position02=position01+trans0; position02(4)=1;
position0=position02*[[1 0 0 0]' [0 1 0 0]' [0 0 1 0]' [-p01(1) -p01(2) -p01(3) 1]']'...
    *[[1 0 0 0]' [0 cos(a1x) sin(a1x) 0]' [0 -sin(a1x) cos(a1x) 0]' [0 0 0 1]']'*[[cos(a1y) 0 -sin(a1y) 0]' [0 1 0 0]'  [sin(a1y) 0 cos(a1y) 0]' [0 0 0 1]']'...
    *[[cos(-q1-theta02) sin(-q1-theta02) 0 0]' [-sin(-q1-theta02) cos(-q1-theta02) 0 0]' [0 0 1 0]' [0 0 0 1]']'...
    *[[cos(-a1y) 0 -sin(-a1y) 0]' [0 1 0 0]'  [sin(-a1y) 0 cos(-a1y) 0]' [0 0 0 1]']'*[[1 0 0 0]' [0 cos(-a1x) sin(-a1x) 0]' [0 -sin(-a1x) cos(-a1x) 0]' [0 0 0 1]']'...
    *[[1 0 0 0]' [0 1 0 0]' [0 0 1 0]' [p01(1) p01(2) p01(3) 1]']';
position0=position0(1:3);
p0=position0;
xx=p0(1);
yy=p0(2);
zz=p0(3);

== matlab function xhand_sphere_tube_r50_v3/contact position imcp  ==
  data: x input; xx output; y input; z input; q1 input; yy output; zz output; l output
function [xx,yy,zz,l] = fcn(x,y,z,q1)

%在食指坐标系下的坐标值
xx1=0+x;
yy1=y*cos(q1);
zz=y*sin(q1);

%在与中指坐标系的平行系下的坐标值
alpha=atan(yy1/xx1);
l=norm([xx1,yy1]);
xx2=l*cos(alpha-4*pi/180);
yy2=l*sin(alpha-4*pi/180);

%在种植坐标系下的坐标值
xx=xx2+18.4272*cos(4*pi/180)-1.2;
yy=yy2-18.4272*sin(4*pi/180)+7.5;
zz=zz+8.5;

l=z;

== matlab function xhand_sphere_tube_r50_v3/contact position rmcp ==
  data: x input; xx output; y input; z input; q1 input; yy output; zz output; l output
function [xx,yy,zz,l] = fcn(x,y,z,q1)

%在食指坐标系下的坐标值
xx1=0+x;
yy1=y*cos(q1);
zz=y*sin(q1);

%在与中指坐标系的平行系下的坐标值
alpha=atan(yy1/xx1);
l=norm([xx1,yy1]);
xx2=l*cos(alpha+3.5*pi/180);
yy2=l*sin(alpha+3.5*pi/180);

%在种植坐标系下的坐标值
xx=xx2-15.9255*cos(3.5*pi/180)-1.2;
yy=yy2-15.9255*sin(3.5*pi/180)+7.5;
zz=zz+8.5;

l=z;

== matlab function xhand_sphere_tube_r50_v3/contact position lmcp ==
  data: x input; xx output; y input; z input; q1 input; yy output; zz output; l output
function [xx,yy,zz,l] = fcn(x,y,z,q1)

%在食指坐标系下的坐标值
xx1=0+x;
yy1=y*cos(q1);
zz=y*sin(q1);

%在与中指坐标系的平行系下的坐标值
alpha=atan(yy1/xx1);
l=norm([xx1,yy1]);
xx2=l*cos(alpha+7*pi/180);
yy2=l*sin(alpha+7*pi/180);

%在种植坐标系下的坐标值
xx=xx2-38.4871*cos(7*pi/180)-1.2;
yy=yy2-38.4871*sin(7*pi/180)+7.5;
zz=zz+8.5;

l=z;

== matlab function xhand_sphere_tube_r50_v3/contact position mmcp ==
  data: x input; xx output; y input; z input; q1 input; yy output; zz output; l output
function [xx,yy,zz,l] = fcn(x,y,z,q1)

xx=0+x;
yy=y*cos(q1);
zz=y*sin(q1);

xx=xx-1.2;
yy=yy+7.5;
zz=zz+8.5;

l=z;

== matlab function xhand_sphere_tube_r50_v3/jacobi mpip ==
  data: y input; r21 input; j output; r22 input
function j = fcn(y,r21,r22)
j11=0;
j12=- (4337*sin(r21))/100000 - sin(r21 + r22)*conj(y);
j13=(4337*cos(r21))/100000 + cos(r21 + r22)*conj(y);
j21=0;
j22=-sin(r21 + r22)*conj(1000*y);
j23=cos(r21 + r22)*conj(1000*y);

j=[[j11 j21];[j12 j22];[j13 j23]];

== matlab function xhand_sphere_tube_r50_v3/jacobi rpip ==
  data: y input; r31 input; j output; r32 input
function j = fcn(y,r31,r32)
j11=(33213302860281518901*sin(r31))/14411518807585587200000 + (8793567079767413*sin(r31 + r32)*conj(y))/144115188075855872;
j12=- (16978400685651381279*sin(r31))/450359962737049600000 - (4495208018440927*sin(r31 + r32)*conj(y))/4503599627370496;
j13=(3777*cos(r31))/100000 + cos(r31 + r32)*conj(y);
j21=(8793567079767413*sin(r31 + r32)*conj(y))/144115188075855872;
j22=-(4495208018440927*sin(r31 + r32)*conj(y))/4503599627370496;
j23=cos(r31 + r32)*conj(y);

j=[[j11 j21];[j12 j22];[j13 j23]];

== matlab function xhand_sphere_tube_r50_v3/jacobi lpip ==
  data: y input; r41 input; j output; r42 input
function j = fcn(y,r41,r42)
j11=(1218711710313245217*sin(r41))/360287970189639680000 + (2194295481298605*sin(r41 + r42)*conj(y))/18014398509481984;
j12=- (993069521325547407*sin(r41))/36028797018963968000 - (8940128928029775*sin(r41 + r42)*conj(y))/9007199254740992;
j13=(2777*cos(r41))/100000 + cos(r41 + r42)*conj(y);
j21=(2194295481298605*sin(r41 + r42)*conj(y))/18014398509481984;
j22=-(8940128928029775*sin(r41 + r42)*conj(y))/9007199254740992;
j23=cos(r41 + r42)*conj(y);

j=[[j11 j21];[j12 j22];[j13 j23]];

== matlab function xhand_sphere_tube_r50_v3/jacobi ipip ==
  data: y input; r11 input; j output; r12 input
function j = fcn(y,r11,r12)
j11=- (4743854959423704813*sin(r11))/1801439850948198400000 - (1255984897914669*sin(r11 + r12)*conj(y))/18014398509481984;
j12=- (33937404077533042611*sin(r11))/900719925474099200000 - (8985280401782643*sin(r11 + r12)*conj(y))/9007199254740992;
j13=(3777*cos(r11))/100000 + cos(r11 + r12)*conj(y);
j21=-(1255984897914669*sin(r11 + r12)*conj(y))/18014398509481984;
j22=-(8985280401782643*sin(r11 + r12)*conj(y))/9007199254740992;
j23=cos(r11 + r12)*conj(y);

j=[[j11 j21];[j12 j22];[j13 j23]];

== matlab function xhand_sphere_tube_r50_v3/jacobi lmcp ==
  data: y input; r41 input; j output
function j  = fcn(y,r41)
j11=(2194295481298605*conj(y)*sin(r41))/18014398509481984;
j12=-(8940128928029775*conj(y)*sin(r41))/9007199254740992;
j13=cos(r41)*conj(y);
j21=0;
j22=0;
j23=0;

j=[[j11 j21];[j12 j22];[j13 j23]];

== matlab function xhand_sphere_tube_r50_v3/jacobi mmcp ==
  data: y input; r21 input; j output
function j = fcn(y,r21)
j11=0;
j12=-conj(y)*sin(r21);
j13=cos(r21)*conj(y);
j21=0;
j22=0;
j23=0;

j=[[j11 j21];[j12 j22];[j13 j23]];

== matlab function xhand_sphere_tube_r50_v3/jacobi imcp ==
  data: y input; r11 input; j output
function j = fcn(y,r11)
j11=-(1255984897914669*conj(y)*sin(r11))/18014398509481984;
j12=-(8985280401782643*conj(y)*sin(r11))/9007199254740992;
j13=cos(r11)*conj(y);
j21=0;
j22=0;
j23=0;

j=[[j11 j21];[j12 j22];[j13 j23]];

== matlab function xhand_sphere_tube_r50_v3/jacobi rmcp ==
  data: y input; r31 input; j output
function j = fcn(y,r31)
j11=(8793567079767413*conj(y)*sin(r31))/144115188075855872;
j12=-(4495208018440927*conj(y)*sin(r31))/4503599627370496;
j13=cos(r31)*conj(y);
j21=0;
j22=0;
j23=0;

j=[[j11 j21];[j12 j22];[j13 j23]];

== matlab function xhand_sphere_tube_r50_v3/jacobi lmcp1 ==
  data: j1 input; j output; j2 input; j3 input; j4 input
function j = fcn(j1,j2,j3,j4)
j=blkdiag(j1,j2,j3,j4);

== matlab function xhand_sphere_tube_r50_v3/jacobi i ==
  data: j1 input; j output; j2 input
function j = fcn(j1,j2)
j=[j1;j2];

== matlab function xhand_sphere_tube_r50_v3/jacobi m ==
  data: j1 input; j output; j2 input
function j = fcn(j1,j2)
j=[j1;j2];

== matlab function xhand_sphere_tube_r50_v3/jacobi r ==
  data: j1 input; j output; j2 input
function j = fcn(j1,j2)
j=[j1;j2];

== matlab function xhand_sphere_tube_r50_v3/jacobi l ==
  data: j1 input; j output; j2 input
function j = fcn(j1,j2)
j=[j1;j2];

== matlab function xhand_sphere_tube_r50_v3/jacobi lmcp2 ==
  data: j input; t11 output; f input; t12 output; t21 output; t22 output; t31 output; t32 output; t41 output; t42 output; q input
function [t11,t12,t21,t22,t31,t32,t41,t42] = fcn(j,f,q)

%用接触力的大小和方向求接触力的旋量

theta=3.14/180*[-4 0 3.5 7];    %四指安装孔处之间的角度（与中指）
dir11=[sin(theta(1))*sin(q(1)) -cos(theta(1))*sin(q(1)) cos(q(1))]';
dir21=[sin(theta(2))*sin(q(3)) -cos(theta(2))*sin(q(3)) cos(q(2))]';
dir31=[sin(theta(3))*sin(q(5)) -cos(theta(3))*sin(q(5)) cos(q(3))]';
dir41=[sin(theta(4))*sin(q(7)) -cos(theta(4))*sin(q(7)) cos(q(4))]';
dir12=[sin(theta(1))*sin(q(1)+q(2)) -cos(theta(1))*sin(q(1)+q(2)) cos(q(1)+q(2))]';
dir22=[sin(theta(2))*sin(q(2)+q(4)) -cos(theta(2))*sin(q(2)+q(4)) cos(q(2)+q(4))]';
dir32=[sin(theta(3))*sin(q(3)+q(6)) -cos(theta(3))*sin(q(3)+q(6)) cos(q(3)+q(6))]';
dir42=[sin(theta(4))*sin(q(4)+q(8)) -cos(theta(4))*sin(q(4)+q(8)) cos(q(4)+q(8))]';

ff=[f(1)*dir11;f(2)*dir12;f(3)*dir21;f(4)*dir22;f(5)*dir31;f(6)*dir32;f(7)*dir41;f(8)*dir42];

%t=J'*f
t=j'*ff;
t11=t(1);
t12=t(2);
t21=t(3);
t22=t(4);
t31=t(5);
t32=t(6);
t41=t(7);
t42=t(8);

== matlab function xhand_sphere_tube_r50_v3/MATLAB Function2 ==
  data: x1 output; x2 output; x3 output; x4 output; k input; t input
function [x1,x2,x3,x4] = fcn(k,t)
r=[[5.1 4.1 6.4 3.3];[3.9 3.9 4.7 3.3];[4.4 4.4 4.4 3.3];[4.3 4.3 4 3.3]]*10^-3;
x=zeros(1,4);
for i=1:4
    x(i)=(r(i,3)*t(2*i-1)+r(i,1)*t(2*i))/((r(i,3)*r(i,2)+r(i,1)*r(i,4))*k);
end
x1=x(1);
x2=x(2);
x3=x(3);
x4=x(4);
